simulink model "MSDR_v1"  (R2018a)
settings: Solver=ode23tb  StartTime=0.0  StopTime=50000  RelTol=1e-3
values from neighbouring files (symbols this model uses):
  a_f = -3.22E-5    (= -3.22e-05)    [MSDR_parameters.m]
  a_g = +2.35E-5    (= 2.35e-05)    [MSDR_parameters.m]
  beta = [0.000223, 0.001457, 0.001307, 0.002628, 0.000766, 0.000280]    [MSDR_parameters.m]
  beta_t = sum(beta)    [MSDR_parameters.m]
  Cp_s_shx = 1549.12e-6    (= 0.00154912)    [MSDR_parameters.m]
  Cst = 10    [MSDR_parameters.m]
  dLb = 0    [MSDR_parameters.m]
  dLs = 0    [MSDR_parameters.m]
  dLsc = 0    [MSDR_parameters.m]
  gamma_I = 5.1135e-2    (= 0.051135)    [MSDR_parameters.m]
  gamma_Xe = 1.1628e-2    (= 0.011628)    [MSDR_parameters.m]
  hA_fg = [h_fg*A_fg/2, h_fg*A_fg/2]    [MSDR_parameters.m]
  hA_p_phx1 = h_p_phx*A_p_phx    [MSDR_parameters.m]
  hA_p_phx2 = h_p_phx*A_p_phx    [MSDR_parameters.m]
  hA_p_phx3 = h_p_phx*A_p_phx    [MSDR_parameters.m]
  hA_p_phx4 = h_p_phx*A_p_phx    [MSDR_parameters.m]
  hA_p_phx5 = h_p_phx*A_p_phx    [MSDR_parameters.m]
  hA_p_phx6 = h_p_phx*A_p_phx    [MSDR_parameters.m]
  hA_p_shx1 = h_p_shx*A_p_shx    [MSDR_parameters.m]
  hA_p_shx2 = h_p_shx*A_p_shx    [MSDR_parameters.m]
  hA_p_shx3 = h_p_shx*A_p_shx    [MSDR_parameters.m]
  hA_p_shx4 = h_p_shx*A_p_shx    [MSDR_parameters.m]
  hA_p_shx5 = h_p_shx*A_p_shx    [MSDR_parameters.m]
  hA_p_shx6 = h_p_shx*A_p_shx    [MSDR_parameters.m]
  hA_s_phx1 = h_s_phx*A_s_phx    [MSDR_parameters.m]
  hA_s_phx2 = h_s_phx*A_s_phx    [MSDR_parameters.m]
  hA_s_phx3 = h_s_phx*A_s_phx    [MSDR_parameters.m]
  hA_s_phx4 = h_s_phx*A_s_phx    [MSDR_parameters.m]
  hA_s_phx5 = h_s_phx*A_s_phx    [MSDR_parameters.m]
  hA_s_phx6 = h_s_phx*A_s_phx    [MSDR_parameters.m]
  hA_s_shx1 = h_s_shx*A_s_shx    [MSDR_parameters.m]
  hA_s_shx2 = h_s_shx*A_s_shx    [MSDR_parameters.m]
  hA_s_shx3 = h_s_shx*A_s_shx    [MSDR_parameters.m]
  hA_s_shx4 = h_s_shx*A_s_shx    [MSDR_parameters.m]
  hA_s_shx5 = h_s_shx*A_s_shx    [MSDR_parameters.m]
  hA_s_shx6 = h_s_shx*A_s_shx    [MSDR_parameters.m]
  I_0 = gamma_I*Sig_f_msdr*phi_0/lam_I    (= 4.38204721773e+16)    [MSDR_parameters.m]
  Ifa = [0.25, 0.25]    [MSDR_parameters.m]
  Ifb = [0.25, 0.25]    [MSDR_parameters.m]
  Ig = [0.5, 0.5]    [MSDR_parameters.m]
  J = 1e-6    (= 1e-06)    [MSDR_parameters.m]
  ka = [0.235, 0.235]    [MSDR_parameters.m]
  kb = [0.235, 0.235]    [MSDR_parameters.m]
  kc = 5    [MSDR_parameters.m]
  kga = [0.015, 0.015]    [MSDR_parameters.m]
  kgb = [0.015, 0.015]    [MSDR_parameters.m]
  L = 8.5344    [MSDR_parameters.m]
  Lam = 2.400E-04    (= 0.00024)    [MSDR_parameters.m]
  lam = [0.0124, 0.0305, 0.111, 0.301, 1.14, 3.01]    [MSDR_parameters.m]
  lam_bubl = 2.0e-2    (= 0.02)    [MSDR_parameters.m]
  lam_I = 2.875e-5    (= 2.875e-05)    [MSDR_parameters.m]
  lam_Xe = 2.0916e-5    (= 2.0916e-05)    [MSDR_parameters.m]
  m_3m = W_3*2    (= 8618.207327)    [MSDR_parameters.m]
  m_fm = W_f*2    (= 9978.96)    [MSDR_parameters.m]
  m_sb = 1717    [MSDR_parameters.m]
  mb_cpb = 2.689619410657651e+00    (= 2.68961941066)    [MSDR_parameters.m]
  mcp_fa = mfa*Cp_f    [MSDR_parameters.m]
  mcp_fb = mfb*Cp_f    [MSDR_parameters.m]
  mcp_g = mg*Cp_g    [MSDR_parameters.m]
  mcp_p_phx1 = Cp_p_phx*mp_phx1    [MSDR_parameters.m]
  mcp_p_phx2 = Cp_p_phx*mp_phx2    [MSDR_parameters.m]
  mcp_p_phx3 = Cp_p_phx*mp_phx3    [MSDR_parameters.m]
  mcp_p_phx4 = Cp_p_phx*mp_phx4    [MSDR_parameters.m]
  mcp_p_phx5 = Cp_p_phx*mp_phx5    [MSDR_parameters.m]
  mcp_p_phx6 = Cp_p_phx*mp_phx6    [MSDR_parameters.m]
  mcp_p_shx1 = Cp_p_shx*mp_shx1    [MSDR_parameters.m]
  mcp_p_shx2 = Cp_p_shx*mp_shx2    [MSDR_parameters.m]
  mcp_p_shx3 = Cp_p_shx*mp_shx3    [MSDR_parameters.m]
  mcp_p_shx4 = Cp_p_shx*mp_shx4    [MSDR_parameters.m]
  mcp_p_shx5 = Cp_p_shx*mp_shx5    [MSDR_parameters.m]
  mcp_p_shx6 = Cp_p_shx*mp_shx6    [MSDR_parameters.m]
  mcp_s_phx1 = Cp_s_phx*ms_phx1    [MSDR_parameters.m]
  mcp_s_phx2 = Cp_s_phx*ms_phx2    [MSDR_parameters.m]
  mcp_s_phx3 = Cp_s_phx*ms_phx3    [MSDR_parameters.m]
  mcp_s_phx4 = Cp_s_phx*ms_phx4    [MSDR_parameters.m]
  mcp_s_phx5 = Cp_s_phx*ms_phx5    [MSDR_parameters.m]
  mcp_s_phx6 = Cp_s_phx*ms_phx6    [MSDR_parameters.m]
  mcp_s_shx1 = Cp_s_shx*ms_shx1    [MSDR_parameters.m]
  mcp_s_shx2 = Cp_s_shx*ms_shx1    [MSDR_parameters.m]
  mcp_s_shx3 = Cp_s_shx*ms_shx1    [MSDR_parameters.m]
  mcp_s_shx4 = Cp_s_shx*ms_shx1    [MSDR_parameters.m]
  mcp_s_shx5 = Cp_s_shx*ms_shx1    [MSDR_parameters.m]
  mcp_s_shx6 = Cp_s_shx*ms_shx1    [MSDR_parameters.m]
  mcp_t_phx1 = Cp_t_phx*mt_phx1    [MSDR_parameters.m]
  mcp_t_phx2 = Cp_t_phx*mt_phx2    [MSDR_parameters.m]
  mcp_t_phx3 = Cp_t_phx*mt_phx3    [MSDR_parameters.m]
  mcp_t_phx4 = Cp_t_phx*mt_phx4    [MSDR_parameters.m]
  mcp_t_phx5 = Cp_t_phx*mt_phx5    [MSDR_parameters.m]
  mcp_t_phx6 = Cp_t_phx*mt_phx6    [MSDR_parameters.m]
  mcp_t_shx1 = Cp_t_phx*mt_shx1    [MSDR_parameters.m]
  mcp_t_shx2 = Cp_t_phx*mt_shx2    [MSDR_parameters.m]
  mcp_t_shx3 = Cp_t_phx*mt_shx3    [MSDR_parameters.m]
  mcp_t_shx4 = Cp_t_phx*mt_shx4    [MSDR_parameters.m]
  mcp_t_shx5 = Cp_t_phx*mt_shx5    [MSDR_parameters.m]
  mcp_t_shx6 = Cp_t_phx*mt_shx6    [MSDR_parameters.m]
  mfa = [mass_fn, mass_fn]    [MSDR_parameters.m]
  mfb = [mass_fn, mass_fn]    [MSDR_parameters.m]
  mp_phx1 = [494.7, 494.7, 494.7, 494.7]    [MSDR_parameters.m]
  mp_phx2 = [494.7, 494.7, 494.7, 494.7]    [MSDR_parameters.m]
  mp_phx3 = [494.7, 494.7, 494.7, 494.7]    [MSDR_parameters.m]
  mp_phx4 = [494.7, 494.7, 494.7, 494.7]    [MSDR_parameters.m]
  mp_phx5 = [494.7, 494.7, 494.7, 494.7]    [MSDR_parameters.m]
  mp_phx6 = [494.7, 494.7, 494.7, 494.7]    [MSDR_parameters.m]
  mp_phxm = (Wp_phx1 + Wp_phx2)*1    (= 1663.16)    [MSDR_parameters.m]
  mp_shx1 = [429.3, 429.3, 429.3, 429.3]    [MSDR_parameters.m]
  mp_shx2 = [429.3, 429.3, 429.3, 429.3]    [MSDR_parameters.m]
  mp_shx3 = [429.3, 429.3, 429.3, 429.3]    [MSDR_parameters.m]
  mp_shx4 = [429.3, 429.3, 429.3, 429.3]    [MSDR_parameters.m]
  mp_shx5 = [429.3, 429.3, 429.3, 429.3]    [MSDR_parameters.m]
  mp_shx6 = [429.3, 429.3, 429.3, 429.3]    [MSDR_parameters.m]
  mp_shxm = (Wp_shx1 + Wp_shx2)*1    (= 932.38)    [MSDR_parameters.m]
  ms_phx1 = [1152.5, 1152.5, 1152.5, 1152.5]    [MSDR_parameters.m]
  ms_phx2 = [1152.5, 1152.5, 1152.5, 1152.5]    [MSDR_parameters.m]
  ms_phx3 = [1152.5, 1152.5, 1152.5, 1152.5]    [MSDR_parameters.m]
  ms_phx4 = [1152.5, 1152.5, 1152.5, 1152.5]    [MSDR_parameters.m]
  ms_phx5 = [1152.5, 1152.5, 1152.5, 1152.5]    [MSDR_parameters.m]
  ms_phx6 = [1152.5, 1152.5, 1152.5, 1152.5]    [MSDR_parameters.m]
  ms_phxm = (Ws_phx1 + Ws_phx2)*1    (= 932.38)    [MSDR_parameters.m]
  ms_shx1 = [1861.5, 1861.5, 1861.5, 1861.5]    [MSDR_parameters.m]
  ms_shx2 = [1861.5, 1861.5, 1861.5, 1861.5]    [MSDR_parameters.m]
  ... (+104 more)
undefined symbols (not defined in the file or in its folder): Ak2, As, C0, Cpp, Cps, Cpsc, Cpw, Dit, Dot, hA_p_thx1, hA_p_thx2, hA_p_thx3, hA_s_thx1, hA_s_thx2, hA_s_thx3, hc0, hfg, hfw0, HFW1, hfw10, HFW2, hpw, Hr, hr0, hwb, hws, hwsc, K3, KBHP, KBLP, Lsc, mcp_p_thx1, mcp_p_thx2, mcp_p_thx3, mcp_s_thx1, mcp_s_thx2, mcp_s_thx3, mcp_t_thx1, mcp_t_thx2, mcp_t_thx3, mp_thx1, mp_thx2, mp_thx3, ms_thx1, ms_thx2, ms_thx3, Mstm, nuf, Pp2, Pp3, Pp4, Pp5
libraries: simulink x20, aerolibconvert2 x2
(part 6 of 7)

== system MSDR_v1/HEAT EXCHANGERS/HEAT EXCHANGER LOOP 5/SHX3 HEAT TRANSFER ==
  PRIMARY FLUID INLET TEMPERATURE : Inport
  SECONDARY FLUID INLET TEMPERATURE : Inport  Port=2
  PRIMARY FLOW FRACTION : Inport  Port=3
  PRIMARY HEAT TRANSFER FRACTION : Inport  Port=4
  SECONDARY FLOW FRACTION : Inport  Port=5
  SECONDARY HEAT TRANSFER FRACTION : Inport  Port=6
  Mux : Mux  Inputs=16
      settings: DisplayOption=signals
  To Workspace : ToWorkspace  VariableName=shx3_ht  SampleTime=-1
  Tp1_shx3 : Integrator  InitialCondition=T0_p_shx3(1)
  Tp2_shx3 : Integrator  InitialCondition=T0_p_shx3(2)
  "Tp3_shx3 " : Integrator  InitialCondition=T0_p_shx3(3)
  Tp4_shx3 : Integrator  InitialCondition=T0_p_shx3(4)
  Ts1_shx3 : Integrator  InitialCondition=T0_s_shx3(1)
  Ts2_shx3 : Integrator  InitialCondition=T0_s_shx3(2)
  Ts3_shx3 : Integrator  InitialCondition=T0_s_shx3(3)
  Ts4_shx3 : Integrator  InitialCondition=T0_s_shx3(4)
  Tt1_shx3 : Integrator  InitialCondition=T0_t_shx3(1)
  Tt2_shx3 : Integrator  InitialCondition=T0_t_shx3(2)
  d(Tp1_shx3)/dt : Fcn  Expr=(u[13]*Wp_shx3/mp_shx3(1))*(u[1] - u[3]) + (u[14]*hA_p_shx3(1)/mcp_p_shx3(1))*(u[7] - u[3])
  d(Tp2_shx3)/dt : Fcn  Expr=(u[13]*Wp_shx3/mp_shx3(2))*(u[3] - u[4]) + (u[14]*hA_p_shx3(2)/mcp_p_shx3(2))*(u[7] - u[3])
  d(Tp3_shx3)/dt : Fcn  Expr=(u[13]*Wp_shx3/mp_shx3(3))*(u[4] - u[5]) + (u[14]*hA_p_shx3(3)/mcp_p_shx3(3))*(u[8] - u[5])
  d(Tp4_shx3)/dt : Fcn  Expr=(u[13]*Wp_shx3/mp_shx3(4))*(u[5] - u[6]) + (u[14]*hA_p_shx3(4)/mcp_p_shx3(4))*(u[8] - u[5])
  d(Ts1_shx3)/dt : Fcn  Expr=(u[15]*Ws_shx3/ms_shx3(1))*(u[2] - u[9]) + (u[16]*hA_s_shx3(1)/mcp_s_shx3(1))*(u[8] - u[9])
  d(Ts2_shx3)/dt : Fcn  Expr=(u[15]*Ws_shx3/ms_shx3(2))*(u[9] - u[10]) + (u[16]*hA_s_shx3(2)/mcp_s_shx3(2))*(u[8] - u[9])
  d(Ts3_shx3)/dt : Fcn  Expr=(u[15]*Ws_shx3/ms_shx3(3))*(u[10] - u[11]) + (u[16]*hA_s_shx3(3)/mcp_s_shx3(3))*(u[7] - u[11])
  d(Ts4_shx3)/dt : Fcn  Expr=(u[15]*Ws_shx3/ms_shx3(4))*(u[11] - u[12]) + (u[16]*hA_s_shx3(4)/mcp_s_shx3(4))*(u[7] - u[11])
  d(Tt1_shx3)/dt : Fcn  Expr=(u[14]*(hA_p_shx3(1) + hA_p_shx3(2))/mcp_t_shx3(1))*(u[3] - u[7]) + (u[16]*(hA_s_shx3(1) + hA_s_shx3(2))/mcp_t_shx3(1))*(u[11] - u[7])
  d(Tt2_shx3)/dt : Fcn  Expr=(u[14]*(hA_p_shx4(3) + hA_p_shx4(4))/mcp_t_shx4(2))*(u[5] - u[8]) + (u[16]*(hA_s_shx4(3) + hA_s_shx4(4))/mcp_t_shx4(2))*(u[9] - u[8])
  SHX3 TEMPERATURES : Outport
  wires:
  Ts1_shx3/1 -> Mux/9
  Ts2_shx3/1 -> Mux/10
  d(Ts2_shx3)/dt/1 -> Ts2_shx3/1
  d(Tp4_shx3)/dt/1 -> Tp4_shx3/1
  Tt1_shx3/1 -> Mux/7
  d(Tp2_shx3)/dt/1 -> Tp2_shx3/1
  Tp4_shx3/1 -> Mux/6
  d(Tt2_shx3)/dt/1 -> Tt2_shx3/1
  SECONDARY FLUID INLET TEMPERATURE/1 -> Mux/2
  Tt2_shx3/1 -> Mux/8
  Mux/1 -> To Workspace/1, SHX3 TEMPERATURES/1, d(Ts4_shx3)/dt/1, d(Ts3_shx3)/dt/1, d(Ts2_shx3)/dt/1, d(Ts1_shx3)/dt/1, d(Tt2_shx3)/dt/1, d(Tt1_shx3)/dt/1, d(Tp4_shx3)/dt/1, d(Tp3_shx3)/dt/1, d(Tp2_shx3)/dt/1, d(Tp1_shx3)/dt/1
  d(Tp1_shx3)/dt/1 -> Tp1_shx3/1
  d(Ts4_shx3)/dt/1 -> Ts4_shx3/1
  Tp1_shx3/1 -> Mux/3
  d(Ts1_shx3)/dt/1 -> Ts1_shx3/1
  d(Ts3_shx3)/dt/1 -> Ts3_shx3/1
  Ts3_shx3/1 -> Mux/11
  Ts4_shx3/1 -> Mux/12
  "Tp3_shx3 "/1 -> Mux/5
  d(Tp3_shx3)/dt/1 -> "Tp3_shx3 "/1
  Tp2_shx3/1 -> Mux/4
  d(Tt1_shx3)/dt/1 -> Tt1_shx3/1
  PRIMARY FLUID INLET TEMPERATURE/1 -> Mux/1
  PRIMARY FLOW FRACTION/1 -> Mux/13
  PRIMARY HEAT TRANSFER FRACTION/1 -> Mux/14
  SECONDARY FLOW FRACTION/1 -> Mux/15
  SECONDARY HEAT TRANSFER FRACTION/1 -> Mux/16

== system MSDR_v1/HEAT EXCHANGERS/HEAT EXCHANGER LOOP 5/SHX3 MATERIAL TRANSPORT ==
  SHX3 TEMPERATURES : Inport
  wires:
  SHX3 TEMPERATURES/1 -> ?

== system MSDR_v1/HEAT EXCHANGERS/HEAT EXCHANGER LOOP 5/SHX4 HEAT TRANSFER ==
  PRIMARY FLUID INLET TEMPERATURE : Inport
  SECONDARY FLUID INLET TEMPERATURE : Inport  Port=2
  PRIMARY FLOW FRACTION : Inport  Port=3
  PRIMARY HEAT TRANSFER FRACTION : Inport  Port=4
  SECONDARY FLOW FRACTION : Inport  Port=5
  SECONDARY HEAT TRANSFER FRACTION : Inport  Port=6
  Mux : Mux  Inputs=16
      settings: DisplayOption=signals
  To Workspace : ToWorkspace  VariableName=shx4_ht  SampleTime=-1
  Tp1_shx4 : Integrator  InitialCondition=T0_p_shx4(1)
  Tp2_shx4 : Integrator  InitialCondition=T0_p_shx4(2)
  "Tp3_shx4 " : Integrator  InitialCondition=T0_p_shx4(3)
  Tp4_shx4 : Integrator  InitialCondition=T0_p_shx4(4)
  Ts1_shx4 : Integrator  InitialCondition=T0_s_shx4(1)
  Ts2_shx4 : Integrator  InitialCondition=T0_s_shx4(2)
  Ts3_shx4 : Integrator  InitialCondition=T0_s_shx4(3)
  Ts4_shx4 : Integrator  InitialCondition=T0_s_shx4(4)
  Tt1_shx4 : Integrator  InitialCondition=T0_t_shx4(1)
  Tt2_shx4 : Integrator  InitialCondition=T0_t_shx4(2)
  d(Tp1_shx4)/dt : Fcn  Expr=(u[13]*Wp_shx4/mp_shx4(1))*(u[1] - u[3]) + (u[14]*hA_p_shx4(1)/mcp_p_shx4(1))*(u[7] - u[3])
  d(Tp2_shx4)/dt : Fcn  Expr=(u[13]*Wp_shx4/mp_shx4(2))*(u[3] - u[4]) + (u[14]*hA_p_shx4(2)/mcp_p_shx4(2))*(u[7] - u[3])
  d(Tp3_shx4)/dt : Fcn  Expr=(u[13]*Wp_shx4/mp_shx4(3))*(u[4] - u[5]) + (u[14]*hA_p_shx4(3)/mcp_p_shx4(3))*(u[8] - u[5])
  d(Tp4_shx4)/dt : Fcn  Expr=(u[13]*Wp_shx4/mp_shx4(4))*(u[5] - u[6]) + (u[14]*hA_p_shx4(4)/mcp_p_shx4(4))*(u[8] - u[5])
  d(Ts1_shx4)/dt : Fcn  Expr=(u[15]*Ws_shx4/ms_shx4(1))*(u[2] - u[9]) + (u[16]*hA_s_shx4(1)/mcp_s_shx4(1))*(u[8] - u[9])
  d(Ts2_shx4)/dt : Fcn  Expr=(u[15]*Ws_shx4/ms_shx4(2))*(u[9] - u[10]) + (u[16]*hA_s_shx4(2)/mcp_s_shx4(2))*(u[8] - u[9])
  d(Ts3_shx4)/dt : Fcn  Expr=(u[15]*Ws_shx4/ms_shx4(3))*(u[10] - u[11]) + (u[16]*hA_s_shx4(3)/mcp_s_shx4(3))*(u[7] - u[11])
  d(Ts4_shx4)/dt : Fcn  Expr=(u[15]*Ws_shx4/ms_shx4(4))*(u[11] - u[12]) + (u[16]*hA_s_shx4(4)/mcp_s_shx4(4))*(u[7] - u[11])
  d(Tt1_shx4)/dt : Fcn  Expr=(u[14]*(hA_p_shx4(1) + hA_p_shx4(2))/mcp_t_shx4(1))*(u[3] - u[7]) + (u[16]*(hA_s_shx4(1) + hA_s_shx4(2))/mcp_t_shx4(1))*(u[11] - u[7])
  d(Tt2_shx4)/dt : Fcn  Expr=(u[14]*(hA_p_shx4(3) + hA_p_shx4(4))/mcp_t_shx4(2))*(u[5] - u[8]) + (u[16]*(hA_s_shx4(3) + hA_s_shx4(4))/mcp_t_shx4(2))*(u[9] - u[8])
  SHX4 TEMPERATURES : Outport
  wires:
  Ts1_shx4/1 -> Mux/9
  Ts2_shx4/1 -> Mux/10
  d(Ts2_shx4)/dt/1 -> Ts2_shx4/1
  d(Tp4_shx4)/dt/1 -> Tp4_shx4/1
  Tt1_shx4/1 -> Mux/7
  d(Tp2_shx4)/dt/1 -> Tp2_shx4/1
  Tp4_shx4/1 -> Mux/6
  d(Tt2_shx4)/dt/1 -> Tt2_shx4/1
  SECONDARY FLUID INLET TEMPERATURE/1 -> Mux/2
  Tt2_shx4/1 -> Mux/8
  Mux/1 -> To Workspace/1, SHX4 TEMPERATURES/1, d(Ts4_shx4)/dt/1, d(Ts3_shx4)/dt/1, d(Ts2_shx4)/dt/1, d(Ts1_shx4)/dt/1, d(Tt2_shx4)/dt/1, d(Tt1_shx4)/dt/1, d(Tp4_shx4)/dt/1, d(Tp3_shx4)/dt/1, d(Tp2_shx4)/dt/1, d(Tp1_shx4)/dt/1
  d(Tp1_shx4)/dt/1 -> Tp1_shx4/1
  d(Ts4_shx4)/dt/1 -> Ts4_shx4/1
  Tp1_shx4/1 -> Mux/3
  d(Ts1_shx4)/dt/1 -> Ts1_shx4/1
  d(Ts3_shx4)/dt/1 -> Ts3_shx4/1
  Ts3_shx4/1 -> Mux/11
  Ts4_shx4/1 -> Mux/12
  "Tp3_shx4 "/1 -> Mux/5
  d(Tp3_shx4)/dt/1 -> "Tp3_shx4 "/1
  Tp2_shx4/1 -> Mux/4
  d(Tt1_shx4)/dt/1 -> Tt1_shx4/1
  PRIMARY FLUID INLET TEMPERATURE/1 -> Mux/1
  PRIMARY FLOW FRACTION/1 -> Mux/13
  PRIMARY HEAT TRANSFER FRACTION/1 -> Mux/14
  SECONDARY FLOW FRACTION/1 -> Mux/15
  SECONDARY HEAT TRANSFER FRACTION/1 -> Mux/16

== system MSDR_v1/HEAT EXCHANGERS/HEAT EXCHANGER LOOP 5/SHX4 MATERIAL TRANSPORT ==
  SHX4 TEMPERATURES : Inport
  wires:
  SHX4 TEMPERATURES/1 -> ?

== system MSDR_v1/HEAT EXCHANGERS/HEAT EXCHANGER LOOP 5/THX2 HEAT TRANSFER ==
  PRIMARY FLUID INLET TEMPERATURE : Inport
  SECONDARY FLUID INLET TEMPERATURE : Inport  Port=2
  PRIMARY FLOW FRACTION : Inport  Port=3
  PRIMARY HEAT TRANSFER FRACTION : Inport  Port=4
  SECONDARY FLOW FRACTION : Inport  Port=5
  SECONDARY HEAT TRANSFER FRACTION : Inport  Port=6
  Mux : Mux  Inputs=16
      settings: DisplayOption=signals
  To Workspace : ToWorkspace  VariableName=thx2_ht  SampleTime=-1
  Tp1_thx2 : Integrator  InitialCondition=T0_p_thx2(1)
  Tp2_thx2 : Integrator  InitialCondition=T0_p_thx2(2)
  "Tp3_thx2 " : Integrator  InitialCondition=T0_p_thx2(3)
  Tp4_thx2 : Integrator  InitialCondition=T0_p_thx2(4)
  Ts1_thx2 : Integrator  InitialCondition=T0_s_thx2(1)
  Ts2_thx2 : Integrator  InitialCondition=T0_s_thx2(2)
  Ts3_thx2 : Integrator  InitialCondition=T0_s_thx2(3)
  Ts4_thx2 : Integrator  InitialCondition=T0_s_thx2(4)
  Tt1_thx2 : Integrator  InitialCondition=T0_t_thx2(1)
  Tt2_thx2 : Integrator  InitialCondition=T0_t_thx2(2)
  d(Tp1_thx2)/dt : Fcn  Expr=(u[13]*Wp_thx2/mp_thx2(1))*(u[1] - u[3]) + (u[14]*hA_p_thx2(1)/mcp_p_thx2(1))*(u[7] - u[3])
  d(Tp2_thx2)/dt : Fcn  Expr=(u[13]*Wp_thx2/mp_thx2(2))*(u[3] - u[4]) + (u[14]*hA_p_thx2(2)/mcp_p_thx2(2))*(u[7] - u[3])
  d(Tp3_thx2)/dt : Fcn  Expr=(u[13]*Wp_thx2/mp_thx2(3))*(u[4] - u[5]) + (u14]*hA_p_thx2(3)/mcp_p_thx2(3))*(u[8] - u[5])
  d(Tp4_thx2)/dt : Fcn  Expr=(u[13]*Wp_thx2/mp_thx2(4))*(u[5] - u[6]) + (u[14]*hA_p_thx2(4)/mcp_p_thx2(4))*(u[8] - u[5])
  d(Ts1_thx2)/dt : Fcn  Expr=(u[15]*Ws_thx2/ms_thx2(1))*(u[2] - u[9]) + (u[16]*hA_s_thx2(1)/mcp_s_thx2(1))*(u[8] - u[9])
  d(Ts2_thx2)/dt : Fcn  Expr=(u[15]*Ws_thx2/ms_thx2(2))*(u[9] - u[10]) + (u[16]*hA_s_thx2(2)/mcp_s_thx2(2))*(u[8] - u[9])
  d(Ts3_thx2)/dt : Fcn  Expr=(u[15]*Ws_thx2/ms_thx2(3))*(u[10] - u[11]) + (u[16]*hA_s_thx2(3)/mcp_s_thx2(3))*(u[7] - u[11])
  d(Ts4_thx2)/dt : Fcn  Expr=(u[15]*Ws_thx2/ms_thx2(4))*(u[11] - u[12]) + (u[16]*hA_s_thx2(4)/mcp_s_thx2(4))*(u[7] - u[11])
  d(Tt1_thx2)/dt : Fcn  Expr=(u[14]*(hA_p_thx2(1) + hA_p_thx2(2))/mcp_t_thx2(1))*(u[3] - u[7]) + (u[16]*(hA_s_thx2(1) + hA_s_thx2(2))/mcp_t_thx2(1))*(u[11] - u[7])
  d(Tt2_thx2)/dt : Fcn  Expr=(u[14]*(hA_p_thx2(3) + hA_p_thx2(4))/mcp_t_thx2(2))*(u[5] - u[8]) + (u[16]*(hA_s_thx2(3) + hA_s_thx2(4))/mcp_t_thx2(2))*(u[9] - u[8])
  THX2 TEMPERATURES : Outport
  wires:
  Ts1_thx2/1 -> Mux/9
  Ts2_thx2/1 -> Mux/10
  d(Ts2_thx2)/dt/1 -> Ts2_thx2/1
  d(Tp4_thx2)/dt/1 -> Tp4_thx2/1
  Tt1_thx2/1 -> Mux/7
  d(Tp2_thx2)/dt/1 -> Tp2_thx2/1
  Tp4_thx2/1 -> Mux/6
  d(Tt2_thx2)/dt/1 -> Tt2_thx2/1
  SECONDARY FLUID INLET TEMPERATURE/1 -> Mux/2
  Tt2_thx2/1 -> Mux/8
  Mux/1 -> To Workspace/1, THX2 TEMPERATURES/1, d(Ts4_thx2)/dt/1, d(Ts3_thx2)/dt/1, d(Ts2_thx2)/dt/1, d(Ts1_thx2)/dt/1, d(Tt2_thx2)/dt/1, d(Tt1_thx2)/dt/1, d(Tp4_thx2)/dt/1, d(Tp3_thx2)/dt/1, d(Tp2_thx2)/dt/1, d(Tp1_thx2)/dt/1
  d(Tp1_thx2)/dt/1 -> Tp1_thx2/1
  d(Ts4_thx2)/dt/1 -> Ts4_thx2/1
  Tp1_thx2/1 -> Mux/3
  d(Ts1_thx2)/dt/1 -> Ts1_thx2/1
  d(Ts3_thx2)/dt/1 -> Ts3_thx2/1
  Ts3_thx2/1 -> Mux/11
  Ts4_thx2/1 -> Mux/12
  "Tp3_thx2 "/1 -> Mux/5
  d(Tp3_thx2)/dt/1 -> "Tp3_thx2 "/1
  Tp2_thx2/1 -> Mux/4
  d(Tt1_thx2)/dt/1 -> Tt1_thx2/1
  PRIMARY FLUID INLET TEMPERATURE/1 -> Mux/1
  PRIMARY FLOW FRACTION/1 -> Mux/13
  PRIMARY HEAT TRANSFER FRACTION/1 -> Mux/14
  SECONDARY FLOW FRACTION/1 -> Mux/15
  SECONDARY HEAT TRANSFER FRACTION/1 -> Mux/16

== system MSDR_v1/HEAT EXCHANGERS/HEAT EXCHANGER LOOP 5/THX2 MATERIAL TRANSPORT ==
  THX2 TEMPERATURES : Inport
  wires:
  THX2 TEMPERATURES/1 -> ?

== system MSDR_v1/HEAT EXCHANGERS/HEAT EXCHANGER LOOP 6/BOILER & REHEATER ==
  Coolant Inlet Temp : Inport
  Power Demand (Frac) : Inport  Port=2
  Fcn : Fcn  Commented=on  Expr=u[1] - u[2]*250/((Ws_shx1 + Ws_shx2)*Cp_s_shx)
  Integrator : Integrator  InitialCondition=400
  Mux : Mux  Inputs=3
      settings: DisplayOption=signals
  To Workspace : ToWorkspace  VariableName=msdr_br_mux3  SampleTime=-1
  ddt_t_b = 1/tau_b*(t_bin-t_b)-p_b/mb_cpb : Fcn  Expr=W_sb*(u(1)-u(3))/m_sb - u(2)/mb_cpb
  Coolant Exit Temp : Outport
  wires:
  Coolant Inlet Temp/1 -> Mux/1
  Mux/1 -> ddt_t_b = 1/tau_b*(t_bin-t_b)-p_b/mb_cpb/1, To Workspace/1
  Power Demand (Frac)/1 -> Mux/2
  Integrator/1 -> Coolant Exit Temp/1, Mux/3
  ddt_t_b = 1/tau_b*(t_bin-t_b)-p_b/mb_cpb/1 -> Integrator/1

== system MSDR_v1/HEAT EXCHANGERS/HEAT EXCHANGER LOOP 6/Fractional Power Demand (fractional) ==
  Add : Sum
  Constant : Constant
  Saturation : Saturate  UpperLimit=1  LowerLimit=0.2
  Saturation1 : Saturate  UpperLimit=.8  LowerLimit=0
  Slider : Subsystem  DialogController=hmiCreateDDGDialog  IsWebBlock=on  mask(MWDashboardBlock){webBlockId=9afe0574-93b5-4d2b-9630-def9aae4c12d, webBlockType=slider, ShowInLibBrowser=on, ShowInitialText=on, HMISrcModelName=MSDR_v1}
      mask prompts: webBlockId "WebBlock Id"; webBlockType "WebBlock Type"; HMISrcModelName "Source Model"
      mask help: SimulinkHMI:dialogs:SliderDialogDesc
      mask Help: helpview([docroot '/mapfiles/simulink.map'], 'hmi_slider')
      mask Display:
      | if strcmp(get_param(bdroot(gcb),'BlockDiagramType'), 'library')
      |     image([(matlabroot) '/toolbox/simulink/hmi/icons/Slider.png']);
      | end
  down 1%/min : simulink/Sources/Ramp  slope=-0.01/60  start=2500  InitialOutput=1
  up 1%/min1 : simulink/Sources/Ramp  slope=0.01/60  start=2500+3600+5000  InitialOutput=0
  Power Demand(frac) : Outport
  wires:
  down 1%/min/1 -> Saturation/1
  Saturation/1 -> Add/1
  up 1%/min1/1 -> Saturation1/1
  Saturation1/1 -> Add/2
  Constant/1 -> Power Demand(frac)/1

== system MSDR_v1/HEAT EXCHANGERS/HEAT EXCHANGER LOOP 6/PHX PRIM MIXING ==
  Tp_phx5 : Inport
  Tp_phx6 : Inport  Port=2
  p_flow_frac : Inport  Port=3
  Fcn : Fcn  Expr=u[3]*Wp_phx5/mp_phxm*(u[1]-u[4]) + u[3]*Wp_phx6/mp_phxm*(u[2]-u[4])
  Integrator : Integrator  InitialCondition=Tf_in
  Mux : Mux
  Tp_phx_mix : Outport
  wires:
  Tp_phx5/1 -> Mux/1
  Tp_phx6/1 -> Mux/2
  Mux/1 -> Fcn/1
  p_flow_frac/1 -> Mux/3
  Fcn/1 -> Integrator/1
  Integrator/1 -> Tp_phx_mix/1, Mux/4

== system MSDR_v1/HEAT EXCHANGERS/HEAT EXCHANGER LOOP 6/PHX SEC MIXING ==
  Ts_phx5 : Inport
  Ts_phx6 : Inport  Port=2
  s_flow_frac : Inport  Port=3
  Fcn : Fcn  Expr=u[3]*Ws_phx5/ms_phxm*(u[1]-u[4]) + u[3]*Ws_phx6/ms_phxm*(u[2]-u[4])
  Integrator : Integrator  InitialCondition=T0_s_phx1(4)
  Mux : Mux
  Ts_phx_mix : Outport
  wires:
  Ts_phx5/1 -> Mux/1
  Ts_phx6/1 -> Mux/2
  Mux/1 -> Fcn/1
  s_flow_frac/1 -> Mux/3
  Fcn/1 -> Integrator/1
  Integrator/1 -> Ts_phx_mix/1, Mux/4

== system MSDR_v1/HEAT EXCHANGERS/HEAT EXCHANGER LOOP 6/PHX//SHX PUMP ==
  1-D Lookup Table : Lookup_n-D  NumberOfTableDimensions=1  BreakpointsForDimension1=xdat  Table=ydat  InternalRulePriority=Speed  RndMeth=Simplest  InputSameDT=on
  Clock : Clock
  Fcn : Fcn  Expr=exp((1/tau_p)*u)
  Final convection flow rate : Constant  Value=therm_conv
  Scope : Scope
  Subtract : Sum  Inputs=-+
  Switch : Switch  Criteria=u2 > Threshold
  Transport Delay : TransportDelay  DelayTime=10000000  InitialOutput=1
  FLOW FRACTION : Outport
  HEAT TRANSFER FRACTION : Outport  Port=2
  wires:
  Transport Delay/1 -> 1-D Lookup Table/1, Scope/1, FLOW FRACTION/1
  Clock/1 -> Fcn/1
  Switch/1 -> Transport Delay/1
  Fcn/1 -> Subtract/1, Switch/1
  Final convection flow rate/1 -> Subtract/2, Switch/3
  Subtract/1 -> Switch/2
  1-D Lookup Table/1 -> HEAT TRANSFER FRACTION/1

== system MSDR_v1/HEAT EXCHANGERS/HEAT EXCHANGER LOOP 6/PHX5 HEAT TRANSFER ==
  PRIMARY FLUID INLET TEMPERATURE : Inport
  SECONDARY FLUID INLET TEMPERATURE : Inport  Port=2
  PRIMARY FLOW FRACTION : Inport  Port=3
  PRIMARY HEAT TRANSFER FRACTION : Inport  Port=4
  SECONDARY FLOW FRACTION : Inport  Port=5
  SECONDARY HEAT TRANSFER FRACTION : Inport  Port=6
  Mux : Mux  Inputs=16
      settings: DisplayOption=signals
  To Workspace : ToWorkspace  VariableName=phx5_ht  SampleTime=-1
  Tp1_phx5 : Integrator  InitialCondition=T0_p_phx5(1)
  Tp2_phx5 : Integrator  InitialCondition=T0_p_phx5(2)
  "Tp3_phx5 " : Integrator  InitialCondition=T0_p_phx5(3)
  Tp4_phx5 : Integrator  InitialCondition=T0_p_phx5(4)
  Ts1_phx5 : Integrator  InitialCondition=T0_s_phx5(1)
  Ts2_phx5 : Integrator  InitialCondition=T0_s_phx5(2)
  Ts3_phx5 : Integrator  InitialCondition=T0_s_phx5(3)
  Ts4_phx5 : Integrator  InitialCondition=T0_s_phx5(4)
  Tt1_phx5 : Integrator  InitialCondition=T0_t_phx5(1)
  Tt2_phx5 : Integrator  InitialCondition=T0_t_phx5(2)
  d(Tp1_phx5)/dt : Fcn  Expr=(u[13]*Wp_phx5/mp_phx5(1))*(u[1] - u[3]) + (u[14]*hA_p_phx5(1)/mcp_p_phx5(1))*(u[7] - u[3])
  d(Tp2_phx5)/dt : Fcn  Expr=(u[13]*Wp_phx5/mp_phx5(2))*(u[3] - u[4]) + (u[14]*hA_p_phx5(2)/mcp_p_phx5(2))*(u[7] - u[3])
  d(Tp3_phx5)/dt : Fcn  Expr=(u[13]*Wp_phx5/mp_phx5(3))*(u[4] - u[5]) + (u[14]*hA_p_phx5(3)/mcp_p_phx5(3))*(u[8] - u[5])
  d(Tp4_phx5)/dt : Fcn  Expr=(u[13]*Wp_phx5/mp_phx5(4))*(u[5] - u[6]) + (u[14]*hA_p_phx5(4)/mcp_p_phx5(4))*(u[8] - u[5])
  d(Ts1_phx5)/dt : Fcn  Expr=(u[15]*Ws_phx5/ms_phx5(1))*(u[2] - u[9]) + (u[16]*hA_s_phx5(1)/mcp_s_phx5(1))*(u[8] - u[9])
  d(Ts2_phx5)/dt : Fcn  Expr=(u[15]*Ws_phx5/ms_phx5(2))*(u[9] - u[10]) + (u[16]*hA_s_phx5(2)/mcp_s_phx5(2))*(u[8] - u[9])
  d(Ts3_phx5)/dt : Fcn  Expr=(u[15]*Ws_phx5/ms_phx5(3))*(u[10] - u[11]) + (u[16]*hA_s_phx5(3)/mcp_s_phx5(3))*(u[7] - u[11])
  d(Ts4_phx5)/dt : Fcn  Expr=(u[15]*Ws_phx5/ms_phx5(4))*(u[11] - u[12]) + (u[16]*hA_s_phx5(4)/mcp_s_phx5(4))*(u[7] - u[11])
  d(Tt1_phx3)/dt : Fcn  Expr=(u[14]*(hA_p_phx5(1) + hA_p_phx5(2))/mcp_t_phx5(1))*(u[3] - u[7]) + (u[16]*(hA_s_phx5(1) + hA_s_phx5(2))/mcp_t_phx5(1))*(u[11] - u[7])
  d(Tt2_phx5)/dt : Fcn  Expr=(u[14]*(hA_p_phx5(3) + hA_p_phx5(4))/mcp_t_phx5(2))*(u[5] - u[8]) + (u[16]*(hA_s_phx5(3) + hA_s_phx5(4))/mcp_t_phx5(2))*(u[9] - u[8])
  PHX5 TEMPERATURES : Outport
  wires:
  Ts1_phx5/1 -> Mux/9
  Ts2_phx5/1 -> Mux/10
  d(Ts2_phx5)/dt/1 -> Ts2_phx5/1
  d(Tp4_phx5)/dt/1 -> Tp4_phx5/1
  Tt1_phx5/1 -> Mux/7
  d(Tp2_phx5)/dt/1 -> Tp2_phx5/1
  Tp4_phx5/1 -> Mux/6
  d(Tt2_phx5)/dt/1 -> Tt2_phx5/1
  SECONDARY FLUID INLET TEMPERATURE/1 -> Mux/2
  Tt2_phx5/1 -> Mux/8
  Mux/1 -> To Workspace/1, PHX5 TEMPERATURES/1, d(Ts4_phx5)/dt/1, d(Ts3_phx5)/dt/1, d(Ts1_phx5)/dt/1, d(Tt2_phx5)/dt/1, d(Tt1_phx3)/dt/1, d(Tp4_phx5)/dt/1, d(Tp3_phx5)/dt/1, d(Tp2_phx5)/dt/1, d(Tp1_phx5)/dt/1, d(Ts2_phx5)/dt/1
  d(Tp1_phx5)/dt/1 -> Tp1_phx5/1
  d(Ts4_phx5)/dt/1 -> Ts4_phx5/1
  Tp1_phx5/1 -> Mux/3
  d(Ts1_phx5)/dt/1 -> Ts1_phx5/1
  d(Ts3_phx5)/dt/1 -> Ts3_phx5/1
  Ts3_phx5/1 -> Mux/11
  Ts4_phx5/1 -> Mux/12
  "Tp3_phx5 "/1 -> Mux/5
  d(Tp3_phx5)/dt/1 -> "Tp3_phx5 "/1
  Tp2_phx5/1 -> Mux/4
  d(Tt1_phx3)/dt/1 -> Tt1_phx5/1
  PRIMARY FLUID INLET TEMPERATURE/1 -> Mux/1
  PRIMARY FLOW FRACTION/1 -> Mux/13
  PRIMARY HEAT TRANSFER FRACTION/1 -> Mux/14
  SECONDARY FLOW FRACTION/1 -> Mux/15
  SECONDARY HEAT TRANSFER FRACTION/1 -> Mux/16

== system MSDR_v1/HEAT EXCHANGERS/HEAT EXCHANGER LOOP 6/PHX5 MATERIAL TRANSPORT ==
  PHX5 TEMPERATURES : Inport
  wires:
  PHX5 TEMPERATURES/1 -> ?

== system MSDR_v1/HEAT EXCHANGERS/HEAT EXCHANGER LOOP 6/PHX6 HEAT TRANSFER ==
  PRIMARY FLUID INLET TEMPERATURE : Inport
  SECONDARY FLUID INLET TEMPERATURE : Inport  Port=2
  PRIMARY FLOW FRACTION : Inport  Port=3
  PRIMARY HEAT TRANSFER FRACTION : Inport  Port=4
  SECONDARY FLOW FRACTION : Inport  Port=5
  SECONDARY HEAT TRANSFER FRACTION : Inport  Port=6
  Mux : Mux  Inputs=16
      settings: DisplayOption=signals
  To Workspace : ToWorkspace  VariableName=phx6_ht  SampleTime=-1
  Tp1_phx6 : Integrator  InitialCondition=T0_p_phx6(1)
  Tp2_phx6 : Integrator  InitialCondition=T0_p_phx6(2)
  "Tp3_phx6 " : Integrator  InitialCondition=T0_p_phx6(3)
  Tp4_phx6 : Integrator  InitialCondition=T0_p_phx6(4)
  Ts1_phx6 : Integrator  InitialCondition=T0_s_phx6(1)
  Ts2_phx6 : Integrator  InitialCondition=T0_s_phx6(2)
  Ts3_phx6 : Integrator  InitialCondition=T0_s_phx6(3)
  Ts4_phx6 : Integrator  InitialCondition=T0_s_phx6(4)
  Tt1_phx6 : Integrator  InitialCondition=T0_t_phx6(1)
  Tt2_phx6 : Integrator  InitialCondition=T0_t_phx6(2)
  d(Tp1_phx6)/dt : Fcn  Expr=(u[13]*Wp_phx6/mp_phx6(1))*(u[1] - u[3]) + (u[14]*hA_p_phx6(1)/mcp_p_phx6(1))*(u[7] - u[3])
  d(Tp2_phx6)/dt : Fcn  Expr=(u[13]*Wp_phx6/mp_phx6(2))*(u[3] - u[4]) + (u[14]*hA_p_phx6(2)/mcp_p_phx6(2))*(u[7] - u[3])
  d(Tp3_phx6)/dt : Fcn  Expr=(u[13]*Wp_phx6/mp_phx6(3))*(u[4] - u[5]) + (u[14]*hA_p_phx6(3)/mcp_p_phx6(3))*(u[8] - u[5])
  d(Tp4_phx6)/dt : Fcn  Expr=(u[13]*Wp_phx6/mp_phx6(4))*(u[5] - u[6]) + (u[14]*hA_p_phx6(4)/mcp_p_phx6(4))*(u[8] - u[5])
  d(Ts1_phx6)/dt : Fcn  Expr=(u[15]*Ws_phx6/ms_phx6(1))*(u[2] - u[9]) + (u[16]*hA_s_phx6(1)/mcp_s_phx6(1))*(u[8] - u[9])
  d(Ts2_phx6)/dt : Fcn  Expr=(u[15]*Ws_phx6/ms_phx6(2))*(u[9] - u[10]) + (u[16]*hA_s_phx6(2)/mcp_s_phx6(2))*(u[8] - u[9])
  d(Ts3_phx6)/dt : Fcn  Expr=(u[15]*Ws_phx6/ms_phx6(3))*(u[10] - u[11]) + (u[16]*hA_s_phx6(3)/mcp_s_phx6(3))*(u[7] - u[11])
  d(Ts4_phx6)/dt : Fcn  Expr=(u[15]*Ws_phx6/ms_phx6(4))*(u[11] - u[12]) + (u[16]*hA_s_phx6(4)/mcp_s_phx6(4))*(u[7] - u[11])
  d(Tt1_phx6)/dt : Fcn  Expr=(u[14]*(hA_p_phx6(1) + hA_p_phx6(2))/mcp_t_phx6(1))*(u[3] - u[7]) + (u[16]*(hA_s_phx6(1) + hA_s_phx6(2))/mcp_t_phx6(1))*(u[11] - u[7])
  d(Tt2_phx6)/dt : Fcn  Expr=(u[14]*(hA_p_phx6(3) + hA_p_phx6(4))/mcp_t_phx6(2))*(u[5] - u[8]) + (u[16]*(hA_s_phx6(3) + hA_s_phx6(4))/mcp_t_phx6(2))*(u[9] - u[8])
  PHX6 TEMPERATURES : Outport
  wires:
  Ts1_phx6/1 -> Mux/9
  Ts2_phx6/1 -> Mux/10
  d(Ts2_phx6)/dt/1 -> Ts2_phx6/1
  d(Tp4_phx6)/dt/1 -> Tp4_phx6/1
  Tt1_phx6/1 -> Mux/7
  d(Tp2_phx6)/dt/1 -> Tp2_phx6/1
  Tp4_phx6/1 -> Mux/6
  d(Tt2_phx6)/dt/1 -> Tt2_phx6/1
  SECONDARY FLUID INLET TEMPERATURE/1 -> Mux/2
  Tt2_phx6/1 -> Mux/8
  Mux/1 -> To Workspace/1, PHX6 TEMPERATURES/1, d(Ts4_phx6)/dt/1, d(Ts3_phx6)/dt/1, d(Ts1_phx6)/dt/1, d(Tt2_phx6)/dt/1, d(Tt1_phx6)/dt/1, d(Tp4_phx6)/dt/1, d(Tp3_phx6)/dt/1, d(Tp2_phx6)/dt/1, d(Tp1_phx6)/dt/1, d(Ts2_phx6)/dt/1
  d(Tp1_phx6)/dt/1 -> Tp1_phx6/1
  d(Ts4_phx6)/dt/1 -> Ts4_phx6/1
  Tp1_phx6/1 -> Mux/3
  d(Ts1_phx6)/dt/1 -> Ts1_phx6/1
  d(Ts3_phx6)/dt/1 -> Ts3_phx6/1
  Ts3_phx6/1 -> Mux/11
  Ts4_phx6/1 -> Mux/12
  "Tp3_phx6 "/1 -> Mux/5
  d(Tp3_phx6)/dt/1 -> "Tp3_phx6 "/1
  Tp2_phx6/1 -> Mux/4
  d(Tt1_phx6)/dt/1 -> Tt1_phx6/1
  PRIMARY FLUID INLET TEMPERATURE/1 -> Mux/1
  SECONDARY FLOW FRACTION/1 -> Mux/15
  PRIMARY HEAT TRANSFER FRACTION/1 -> Mux/14
  PRIMARY FLOW FRACTION/1 -> Mux/13
  SECONDARY HEAT TRANSFER FRACTION/1 -> Mux/16

== system MSDR_v1/HEAT EXCHANGERS/HEAT EXCHANGER LOOP 6/PHX6 MATERIAL TRANSPORT ==
  PHX6 TEMPERATURES : Inport
  wires:
  PHX6 TEMPERATURES/1 -> ?

== system MSDR_v1/HEAT EXCHANGERS/HEAT EXCHANGER LOOP 6/SHX PRIM MIXING ==
  Tp_shx5 : Inport
  Tp_shx6 : Inport  Port=2
  p_flow_frac : Inport  Port=3
  Fcn : Fcn  Expr=u[3]*Wp_shx5/mp_shxm*(u[1]-u[4]) + u[3]*Wp_shx6/mp_shxm*(u[2]-u[4])
  Integrator : Integrator  InitialCondition=T0_p_shx1(4)
  Mux : Mux
  Tp_shx_mix : Outport
  wires:
  Tp_shx5/1 -> Mux/1
  Tp_shx6/1 -> Mux/2
  Mux/1 -> Fcn/1
  p_flow_frac/1 -> Mux/3
  Fcn/1 -> Integrator/1
  Integrator/1 -> Tp_shx_mix/1, Mux/4

== system MSDR_v1/HEAT EXCHANGERS/HEAT EXCHANGER LOOP 6/SHX SEC MIXING ==
  Ts_shx5 : Inport
  Ts_shx6 : Inport  Port=2
  s_flow_frac : Inport  Port=3
  Fcn : Fcn  Expr=u[3]*Ws_shx5/ms_shxm*(u[1]-u[4]) + u[3]*Ws_shx6/ms_shxm*(u[2]-u[4])
  Integrator : Integrator  InitialCondition=T0_s_shx1(4)
  Mux : Mux
  Ts_shx_mix : Outport
  wires:
  Ts_shx5/1 -> Mux/1
  Ts_shx6/1 -> Mux/2
  Mux/1 -> Fcn/1
  s_flow_frac/1 -> Mux/3
  Fcn/1 -> Integrator/1
  Integrator/1 -> Ts_shx_mix/1, Mux/4

== system MSDR_v1/HEAT EXCHANGERS/HEAT EXCHANGER LOOP 6/SHX//THX PUMP ==
  1-D Lookup Table : Lookup_n-D  NumberOfTableDimensions=1  BreakpointsForDimension1=xdat  Table=ydat  InternalRulePriority=Speed  RndMeth=Simplest  InputSameDT=on
  Clock : Clock
  Fcn : Fcn  Expr=exp((1/tau_p)*u)
  Final convection flow rate : Constant  Value=therm_conv
  Scope : Scope
  Subtract : Sum  Inputs=-+
  Switch : Switch  Criteria=u2 > Threshold
  Transport Delay : TransportDelay  DelayTime=20000000  InitialOutput=1
  FLOW FRACTION : Outport
  HEAT TRANSFER FRACTION : Outport  Port=2
  wires:
  Transport Delay/1 -> 1-D Lookup Table/1, Scope/1, FLOW FRACTION/1
  Clock/1 -> Fcn/1
  Switch/1 -> Transport Delay/1
  Fcn/1 -> Subtract/1, Switch/1
  Final convection flow rate/1 -> Subtract/2, Switch/3
  Subtract/1 -> Switch/2
  1-D Lookup Table/1 -> HEAT TRANSFER FRACTION/1

== system MSDR_v1/HEAT EXCHANGERS/HEAT EXCHANGER LOOP 6/SHX5 HEAT TRANSFER ==
  PRIMARY FLUID INLET TEMPERATURE : Inport
  SECONDARY FLUID INLET TEMPERATURE : Inport  Port=2
  PRIMARY FLOW FRACTION : Inport  Port=3
  PRIMARY HEAT TRANSFER FRACTION : Inport  Port=4
  SECONDARY FLOW FRACTION : Inport  Port=5
  SECONDARY HEAT TRANSFER FRACTION : Inport  Port=6
  Mux : Mux  Inputs=16
      settings: DisplayOption=signals
  To Workspace : ToWorkspace  VariableName=shx5_ht  SampleTime=-1
  Tp1_shx5 : Integrator  InitialCondition=T0_p_shx3(1)
  Tp2_shx5 : Integrator  InitialCondition=T0_p_shx5(2)
  "Tp3_shx5 " : Integrator  InitialCondition=T0_p_shx5(3)
  Tp4_shx5 : Integrator  InitialCondition=T0_p_shx5(4)
  Ts1_shx5 : Integrator  InitialCondition=T0_s_shx5(1)
  Ts2_shx5 : Integrator  InitialCondition=T0_s_shx5(2)
  Ts3_shx5 : Integrator  InitialCondition=T0_s_shx5(3)
  Ts4_shx5 : Integrator  InitialCondition=T0_s_shx5(4)
  Tt1_shx5 : Integrator  InitialCondition=T0_t_shx5(1)
  Tt2_shx5 : Integrator  InitialCondition=T0_t_shx5(2)
  d(Tp1_shx5)/dt : Fcn  Expr=(u[13]*Wp_shx5/mp_shx5(1))*(u[1] - u[3]) + (u[14]*hA_p_shx5(1)/mcp_p_shx5(1))*(u[7] - u[3])
  d(Tp2_shx5)/dt : Fcn  Expr=(u[13]*Wp_shx5/mp_shx5(2))*(u[3] - u[4]) + (u[14]*hA_p_shx5(2)/mcp_p_shx5(2))*(u[7] - u[3])
  d(Tp3_shx5)/dt : Fcn  Expr=(u[13]*Wp_shx5/mp_shx5(3))*(u[4] - u[5]) + (u[14]*hA_p_shx5(3)/mcp_p_shx5(3))*(u[8] - u[5])
  d(Tp4_shx5)/dt : Fcn  Expr=(u[13]*Wp_shx5/mp_shx5(4))*(u[5] - u[6]) + (u[14]*hA_p_shx5(4)/mcp_p_shx5(4))*(u[8] - u[5])
  d(Ts1_shx5)/dt : Fcn  Expr=(u[15]*Ws_shx5/ms_shx5(1))*(u[2] - u[9]) + (u[16]*hA_s_shx5(1)/mcp_s_shx5(1))*(u[8] - u[9])
  d(Ts2_shx5)/dt : Fcn  Expr=(u[15]*Ws_shx5/ms_shx5(2))*(u[9] - u[10]) + (u[16]*hA_s_shx5(2)/mcp_s_shx5(2))*(u[8] - u[9])
  d(Ts3_shx5)/dt : Fcn  Expr=(u[15]*Ws_shx5/ms_shx5(3))*(u[10] - u[11]) + (u[16]*hA_s_shx5(3)/mcp_s_shx5(3))*(u[7] - u[11])
  d(Ts4_shx5)/dt : Fcn  Expr=(u[15]*Ws_shx5/ms_shx5(4))*(u[11] - u[12]) + (u[16]*hA_s_shx5(4)/mcp_s_shx5(4))*(u[7] - u[11])
  d(Tt1_shx5)/dt : Fcn  Expr=(u[14]*(hA_p_shx5(1) + hA_p_shx5(2))/mcp_t_shx5(1))*(u[3] - u[7]) + (u[16]*(hA_s_shx5(1) + hA_s_shx5(2))/mcp_t_shx5(1))*(u[11] - u[7])
  d(Tt2_shx5)/dt : Fcn  Expr=(u[14]*(hA_p_shx5(3) + hA_p_shx5(4))/mcp_t_shx5(2))*(u[5] - u[8]) + (u[16]*(hA_s_shx5(3) + hA_s_shx5(4))/mcp_t_shx5(2))*(u[9] - u[8])
  SHX5 TEMPERATURES : Outport
  wires:
  Ts1_shx5/1 -> Mux/9
  Ts2_shx5/1 -> Mux/10
  d(Ts2_shx5)/dt/1 -> Ts2_shx5/1
  d(Tp4_shx5)/dt/1 -> Tp4_shx5/1
  Tt1_shx5/1 -> Mux/7
  d(Tp2_shx5)/dt/1 -> Tp2_shx5/1
  Tp4_shx5/1 -> Mux/6
  d(Tt2_shx5)/dt/1 -> Tt2_shx5/1
  SECONDARY FLUID INLET TEMPERATURE/1 -> Mux/2
  Tt2_shx5/1 -> Mux/8
  Mux/1 -> To Workspace/1, SHX5 TEMPERATURES/1, d(Ts4_shx5)/dt/1, d(Ts3_shx5)/dt/1, d(Ts2_shx5)/dt/1, d(Ts1_shx5)/dt/1, d(Tt2_shx5)/dt/1, d(Tt1_shx5)/dt/1, d(Tp4_shx5)/dt/1, d(Tp3_shx5)/dt/1, d(Tp2_shx5)/dt/1, d(Tp1_shx5)/dt/1
  d(Tp1_shx5)/dt/1 -> Tp1_shx5/1
  d(Ts4_shx5)/dt/1 -> Ts4_shx5/1
  Tp1_shx5/1 -> Mux/3
  d(Ts1_shx5)/dt/1 -> Ts1_shx5/1
  d(Ts3_shx5)/dt/1 -> Ts3_shx5/1
  Ts3_shx5/1 -> Mux/11
  Ts4_shx5/1 -> Mux/12
  "Tp3_shx5 "/1 -> Mux/5
  d(Tp3_shx5)/dt/1 -> "Tp3_shx5 "/1
  Tp2_shx5/1 -> Mux/4
  d(Tt1_shx5)/dt/1 -> Tt1_shx5/1
  PRIMARY FLUID INLET TEMPERATURE/1 -> Mux/1
  SECONDARY FLOW FRACTION/1 -> Mux/15
  PRIMARY HEAT TRANSFER FRACTION/1 -> Mux/14
  PRIMARY FLOW FRACTION/1 -> Mux/13
  SECONDARY HEAT TRANSFER FRACTION/1 -> Mux/16

== system MSDR_v1/HEAT EXCHANGERS/HEAT EXCHANGER LOOP 6/SHX5 MATERIAL TRANSPORT ==
  SHX5 TEMPERATURES : Inport
  wires:
  SHX5 TEMPERATURES/1 -> ?

== system MSDR_v1/HEAT EXCHANGERS/HEAT EXCHANGER LOOP 6/SHX6 HEAT TRANSFER ==
  PRIMARY FLUID INLET TEMPERATURE : Inport
  SECONDARY FLUID INLET TEMPERATURE : Inport  Port=2
  PRIMARY FLOW FRACTION : Inport  Port=3
  PRIMARY HEAT TRANSFER FRACTION : Inport  Port=4
  SECONDARY FLOW FRACTION : Inport  Port=5
  SECONDARY HEAT TRANSFER FRACTION : Inport  Port=6
  Mux : Mux  Inputs=16
      settings: DisplayOption=signals
  To Workspace : ToWorkspace  VariableName=shx6_ht  SampleTime=-1
  Tp1_shx6 : Integrator  InitialCondition=T0_p_shx6(1)
  Tp2_shx6 : Integrator  InitialCondition=T0_p_shx6(2)
  "Tp3_shx6 " : Integrator  InitialCondition=T0_p_shx6(3)
  Tp4_shx6 : Integrator  InitialCondition=T0_p_shx6(4)
  Ts1_shx6 : Integrator  InitialCondition=T0_s_shx6(1)
  Ts2_shx6 : Integrator  InitialCondition=T0_s_shx6(2)
  Ts3_shx6 : Integrator  InitialCondition=T0_s_shx6(3)
  Ts4_shx6 : Integrator  InitialCondition=T0_s_shx6(4)
  Tt1_shx6 : Integrator  InitialCondition=T0_t_shx6(1)
  Tt2_shx6 : Integrator  InitialCondition=T0_t_shx6(2)
  d(Tp1_shx6)/dt : Fcn  Expr=(u[13]*Wp_shx6/mp_shx6(1))*(u[1] - u[3]) + (u[14]*hA_p_shx6(1)/mcp_p_shx6(1))*(u[7] - u[3])
  d(Tp2_shx6)/dt : Fcn  Expr=(u[13]*Wp_shx6/mp_shx6(2))*(u[3] - u[4]) + (u[14]*hA_p_shx6(2)/mcp_p_shx6(2))*(u[7] - u[3])
  d(Tp3_shx6)/dt : Fcn  Expr=(u[13]*Wp_shx6/mp_shx6(3))*(u[4] - u[5]) + (u[14]*hA_p_shx6(3)/mcp_p_shx6(3))*(u[8] - u[5])
  d(Tp4_shx6)/dt : Fcn  Expr=(u[13]*Wp_shx6/mp_shx6(4))*(u[5] - u[6]) + (u[14]*hA_p_shx6(4)/mcp_p_shx6(4))*(u[8] - u[5])
  d(Ts1_shx6)/dt : Fcn  Expr=(u[15]*Ws_shx6/ms_shx6(1))*(u[2] - u[9]) + (u[16]*hA_s_shx6(1)/mcp_s_shx6(1))*(u[8] - u[9])
  d(Ts2_shx6)/dt : Fcn  Expr=(u[15]*Ws_shx6/ms_shx6(2))*(u[9] - u[10]) + (u[16]*hA_s_shx6(2)/mcp_s_shx6(2))*(u[8] - u[9])
  d(Ts3_shx6)/dt : Fcn  Expr=(u[15]*Ws_shx6/ms_shx6(3))*(u[10] - u[11]) + (u[16]*hA_s_shx6(3)/mcp_s_shx6(3))*(u[7] - u[11])
  d(Ts4_shx4)/dt : Fcn  Expr=(u[15]*Ws_shx6/ms_shx6(4))*(u[11] - u[12]) + (u[16]*hA_s_shx6(4)/mcp_s_shx6(4))*(u[7] - u[11])
  d(Tt1_shx6)/dt : Fcn  Expr=(u[14]*(hA_p_shx6(1) + hA_p_shx6(2))/mcp_t_shx6(1))*(u[3] - u[7]) + (u[16]*(hA_s_shx6(1) + hA_s_shx6(2))/mcp_t_shx6(1))*(u[11] - u[7])
  d(Tt2_shx6)/dt : Fcn  Expr=(u[14]*(hA_p_shx6(3) + hA_p_shx6(4))/mcp_t_shx6(2))*(u[5] - u[8]) + (u[16]*(hA_s_shx6(3) + hA_s_shx6(4))/mcp_t_shx6(2))*(u[9] - u[8])
  SHX6 TEMPERATURES : Outport
  wires:
  Ts1_shx6/1 -> Mux/9
  Ts2_shx6/1 -> Mux/10
  d(Ts2_shx6)/dt/1 -> Ts2_shx6/1
  d(Tp4_shx6)/dt/1 -> Tp4_shx6/1
  Tt1_shx6/1 -> Mux/7
  d(Tp2_shx6)/dt/1 -> Tp2_shx6/1
  Tp4_shx6/1 -> Mux/6
  d(Tt2_shx6)/dt/1 -> Tt2_shx6/1
  SECONDARY FLUID INLET TEMPERATURE/1 -> Mux/2
  Tt2_shx6/1 -> Mux/8
  Mux/1 -> To Workspace/1, SHX6 TEMPERATURES/1, d(Ts4_shx4)/dt/1, d(Ts3_shx6)/dt/1, d(Ts2_shx6)/dt/1, d(Ts1_shx6)/dt/1, d(Tt2_shx6)/dt/1, d(Tt1_shx6)/dt/1, d(Tp4_shx6)/dt/1, d(Tp3_shx6)/dt/1, d(Tp2_shx6)/dt/1, d(Tp1_shx6)/dt/1
  d(Tp1_shx6)/dt/1 -> Tp1_shx6/1
  d(Ts4_shx4)/dt/1 -> Ts4_shx6/1
  Tp1_shx6/1 -> Mux/3
  d(Ts1_shx6)/dt/1 -> Ts1_shx6/1
  d(Ts3_shx6)/dt/1 -> Ts3_shx6/1
  Ts3_shx6/1 -> Mux/11
  Ts4_shx6/1 -> Mux/12
  "Tp3_shx6 "/1 -> Mux/5
  d(Tp3_shx6)/dt/1 -> "Tp3_shx6 "/1
  Tp2_shx6/1 -> Mux/4
  d(Tt1_shx6)/dt/1 -> Tt1_shx6/1
  PRIMARY FLUID INLET TEMPERATURE/1 -> Mux/1
  SECONDARY FLOW FRACTION/1 -> Mux/15
  PRIMARY HEAT TRANSFER FRACTION/1 -> Mux/14
  PRIMARY FLOW FRACTION/1 -> Mux/13
  SECONDARY HEAT TRANSFER FRACTION/1 -> Mux/16

== system MSDR_v1/HEAT EXCHANGERS/HEAT EXCHANGER LOOP 6/SHX6 MATERIAL TRANSPORT ==
  SHX6 TEMPERATURES : Inport
  wires:
  SHX6 TEMPERATURES/1 -> ?

== system MSDR_v1/HEAT EXCHANGERS/HEAT EXCHANGER LOOP 6/THX2 HEAT TRANSFER ==
  PRIMARY FLUID INLET TEMPERATURE : Inport
  SECONDARY FLUID INLET TEMPERATURE : Inport  Port=2
  PRIMARY FLOW FRACTION : Inport  Port=3
  PRIMARY HEAT TRANSFER FRACTION : Inport  Port=4
  SECONDARY FLOW FRACTION : Inport  Port=5
  SECONDARY HEAT TRANSFER FRACTION : Inport  Port=6
  Mux : Mux  Inputs=16
      settings: DisplayOption=signals
  To Workspace : ToWorkspace  VariableName=thx3_ht  SampleTime=-1
  Tp1_thx3 : Integrator  InitialCondition=T0_p_thx3(1)
  Tp2_thx3 : Integrator  InitialCondition=T0_p_thx3(2)
  "Tp3_thx3 " : Integrator  InitialCondition=T0_p_thx3(3)
  Tp4_thx3 : Integrator  InitialCondition=T0_p_thx3(4)
  Ts1_thx3 : Integrator  InitialCondition=T0_s_thx3(1)
  Ts2_thx3 : Integrator  InitialCondition=T0_s_thx3(2)
  Ts3_thx3 : Integrator  InitialCondition=T0_s_thx3(3)
  Ts4_thx3 : Integrator  InitialCondition=T0_s_thx3(4)
  Tt1_thx3 : Integrator  InitialCondition=T0_t_thx3(1)
  Tt2_thx3 : Integrator  InitialCondition=T0_t_thx3(2)
  d(Tp1_thx3)/dt : Fcn  Expr=(u[13]*Wp_thx3/mp_thx3(1))*(u[1] - u[3]) + (u[14]*hA_p_thx3(1)/mcp_p_thx3(1))*(u[7] - u[3])
  d(Tp2_thx3)/dt : Fcn  Expr=(u[13]*Wp_thx3/mp_thx3(2))*(u[3] - u[4]) + (u[14]*hA_p_thx3(2)/mcp_p_thx3(2))*(u[7] - u[3])
  d(Tp3_thx3)/dt : Fcn  Expr=(u[13]*Wp_thx3/mp_thx3(3))*(u[4] - u[5]) + (u[14]*hA_p_thx3(3)/mcp_p_thx3(3))*(u[8] - u[5])
  d(Tp4_thx3)/dt : Fcn  Expr=(u[13]*Wp_thx3/mp_thx3(4))*(u[5] - u[6]) + (u[14]*hA_p_thx3(4)/mcp_p_thx3(4))*(u[8] - u[5])
  d(Ts1_thx3)/dt : Fcn  Expr=(u[15]*Ws_thx3/ms_thx3(1))*(u[2] - u[9]) + (u[16]*hA_s_thx3(1)/mcp_s_thx3(1))*(u[8] - u[9])
  d(Ts2_thx3)/dt : Fcn  Expr=(u[15]*Ws_thx3/ms_thx3(2))*(u[9] - u[10]) + (u[16]*hA_s_thx3(2)/mcp_s_thx3(2))*(u[8] - u[9])
  d(Ts3_thx3)/dt : Fcn  Expr=(u[15]*Ws_thx3/ms_thx3(3))*(u[10] - u[11]) + (u[16]*hA_s_thx3(3)/mcp_s_thx3(3))*(u[7] - u[11])
  d(Ts4_thx3)/dt : Fcn  Expr=(u[15]*Ws_thx3/ms_thx3(4))*(u[11] - u[12]) + (u[16]*hA_s_thx3(4)/mcp_s_thx3(4))*(u[7] - u[11])
  d(Tt1_thx3)/dt : Fcn  Expr=(u[14]*(hA_p_thx3(1) + hA_p_thx3(2))/mcp_t_thx3(1))*(u[3] - u[7]) + (u[16]*(hA_s_thx3(1) + hA_s_thx3(2))/mcp_t_thx3(1))*(u[11] - u[7])
  d(Tt2_thx3)/dt : Fcn  Expr=(u[14]*(hA_p_thx3(3) + hA_p_thx3(4))/mcp_t_thx3(2))*(u[5] - u[8]) + (u[16]*(hA_s_thx3(3) + hA_s_thx3(4))/mcp_t_thx3(2))*(u[9] - u[8])
  THX3 TEMPERATURES : Outport
  wires:
  Ts1_thx3/1 -> Mux/9
  Ts2_thx3/1 -> Mux/10
  d(Ts2_thx3)/dt/1 -> Ts2_thx3/1
  d(Tp4_thx3)/dt/1 -> Tp4_thx3/1
  Tt1_thx3/1 -> Mux/7
  d(Tp2_thx3)/dt/1 -> Tp2_thx3/1
  Tp4_thx3/1 -> Mux/6
  d(Tt2_thx3)/dt/1 -> Tt2_thx3/1
  SECONDARY FLUID INLET TEMPERATURE/1 -> Mux/2
  Tt2_thx3/1 -> Mux/8
  Mux/1 -> To Workspace/1, THX3 TEMPERATURES/1, d(Ts4_thx3)/dt/1, d(Ts3_thx3)/dt/1, d(Ts2_thx3)/dt/1, d(Ts1_thx3)/dt/1, d(Tt2_thx3)/dt/1, d(Tt1_thx3)/dt/1, d(Tp4_thx3)/dt/1, d(Tp3_thx3)/dt/1, d(Tp2_thx3)/dt/1, d(Tp1_thx3)/dt/1
  d(Tp1_thx3)/dt/1 -> Tp1_thx3/1
  d(Ts4_thx3)/dt/1 -> Ts4_thx3/1
  Tp1_thx3/1 -> Mux/3
  d(Ts1_thx3)/dt/1 -> Ts1_thx3/1
  d(Ts3_thx3)/dt/1 -> Ts3_thx3/1
  Ts3_thx3/1 -> Mux/11
  Ts4_thx3/1 -> Mux/12
  "Tp3_thx3 "/1 -> Mux/5
  d(Tp3_thx3)/dt/1 -> "Tp3_thx3 "/1
  Tp2_thx3/1 -> Mux/4
  d(Tt1_thx3)/dt/1 -> Tt1_thx3/1
  PRIMARY FLUID INLET TEMPERATURE/1 -> Mux/1
  SECONDARY HEAT TRANSFER FRACTION/1 -> Mux/16
  PRIMARY FLOW FRACTION/1 -> Mux/13
  PRIMARY HEAT TRANSFER FRACTION/1 -> Mux/14
  SECONDARY FLOW FRACTION/1 -> Mux/15

== system MSDR_v1/HEAT EXCHANGERS/HEAT EXCHANGER LOOP 6/THX3 MATERIAL TRANSPORT ==
  THX3 TEMPERATURES : Inport
  wires:
  THX3 TEMPERATURES/1 -> ?

== system MSDR_v1/BALANCE OF PLANT/POWER/BOP/H.P. Turbine ==
  note: h2=hc-nhp(hc-h'2)
  note: ((u[6]-u[3])-u[2])/T_w2
  note: ((u[5]-u[9])/eta_hp_isen)+u[9]
  note: 1067+0.37*(PR-200)-0.0011*(PR-200)^2-0.1*(PC-1000)
  note: ((h'2-hc)/eta_hp_isen)+hc
  note: KBHP*u[6]
  note: KBHP*w2
  note: ((w2-wBHP)-w''2)*(1/T_w2)
  note: 1067+0.37*(u[8]/144-200)-0.0011*(u[8]/144-200)^2-0.1*(u[7]/144-1000)
  note: u[9]-0.3*(u[9]-u[5])
  W2 : Inport
  hc : Inport  Port=2
  PC : Inport  Port=3
  PR : Inport  Port=4
  Display1 : Display
  Display20 : Display
  IC5 : InitialCondition  Value=1131
  Mux1 : Mux  Inputs=9
      settings: DisplayOption=signals
  dw''2/dt : Fcn  Expr=((u[6]-u[3])-u[2])/T_w2
  h'2 : Fcn  Expr=1067+0.37*(u[8]/144-200)-0.0011*(u[8]/144-200)^2-0.1*(u[7]/144-1000)
  h2_calc : Fcn  Expr=u[9]-0.3*(u[9]-u[5])
  output : ToWorkspace  VariableName=hpt  SampleTime=-1
  w''2 : Integrator  InitialCondition=w2_hpout
  wBHP : Fcn  Expr=KBHP*u[6]
  W2'' : Outport
  WBHP : Outport  Port=2
  h2 : Outport  Port=3
  wires:
  dw''2/dt/1 -> w''2/1, Mux1/1
  w''2/1 -> W2''/1, Mux1/2
  W2/1 -> Mux1/6
  hc/1 -> Mux1/9
  PC/1 -> Mux1/7
  PR/1 -> Mux1/8
  h2_calc/1 -> Display1/1, h2/1, Mux1/4
  wBHP/1 -> WBHP/1, Mux1/3
  h'2/1 -> Display20/1, Mux1/5
  Mux1/1 -> output/1, IC5/1, wBHP/1, dw''2/dt/1, h'2/1
  IC5/1 -> h2_calc/1

== system MSDR_v1/BALANCE OF PLANT/POWER/BOP/Heater 1 ==
  note: (u[3]/TH1*u[7])+(u[11]-u[2])/TH1
  note: Tco
  note: u(9)+u(13)+u(12)
  note: Wco'+WBLP+W1HP
  note: HFW1*(w1HP+wBLP)
  note: (QH1/(TH1*wfw))+(h0-h1fw)/TH1
  note: HFW1*(u[12]+u[13])
  WBLP : Inport
  Tco : Inport  Port=2
  Wco' : Inport  Port=3
  W1HP : Inport  Port=4
  h0 : Inport  Port=5
  1/Wfw1 : Math  Operator=reciprocal  SaturateOnIntegerOverflow=on
  Fcn : Fcn  Expr=u(10)
  Init1 : InitialCondition  Value=1/Wfw
  Init2 : InitialCondition  Value=Wfw
  Mux1 : Mux  Inputs=13
      settings: DisplayOption=signals
  QH1 : Fcn  Expr=HFW1*(u[12]+u[13])
  Scope{,1..7} (8 alike) : Scope
  Tci : Constant  VectorParams1D=off
  Tci1 : Constant  VectorParams1D=off
  Wfw_calc : Fcn  Expr=u(9)+u(13)+u(12)
  dh1fw/dt : Fcn  Expr=(u[3]/TH1*u[7])+(u[11]-u[2])/TH1
  h1fw_calc : Integrator  InitialCondition=hfw10
  ho : Lookup  InputValues=[162.18,170.00,182.81,193.16,211.95,227.92,240.03]  Table=[130.18 138.02 150.86 161.25 180.16 196.27 208.52]  RndMeth=Nearest  SaturateOnIntegerOverflow=on
  output : ToWorkspace  VariableName=fha  SampleTime=-1
  Wfw_out : Outport
  h1fw : Outport  Port=2
  wires:
  dh1fw/dt/1 -> Mux1/1, h1fw_calc/1, Scope4/1
  h1fw_calc/1 -> Mux1/2, Scope2/1, h1fw/1
  WBLP/1 -> Mux1/13, Scope7/1
  W1HP/1 -> Scope6/1, Mux1/12
  QH1/1 -> Scope1/1, Mux1/3
  Fcn/1 -> ho/1
  ho/1 -> Mux1/8, Scope/1
  1/Wfw1/1 -> Init1/1
  Tco/1 -> Mux1/10
  Wco'/1 -> Scope5/1, Mux1/9
  Wfw_calc/1 -> Init2/1
  Tci1/1 -> Mux1/5
  Tci/1 -> Mux1/4
  Mux1/1 -> Fcn/1, Wfw_calc/1, dh1fw/dt/1, QH1/1, output/1
  Init1/1 -> Scope3/1, Mux1/7
  Init2/1 -> Mux1/6, Wfw_out/1, 1/Wfw1/1
  h0/1 -> Mux1/11

== system MSDR_v1/BALANCE OF PLANT/POWER/BOP/Heater 2 ==
  note: 0.95484181*u[2] + 38.33195608
  note: ((w2-w'2)/TH2P)+((w1PR-w1HP)/TH2P)
  note: HFW2*(wBHP+wMS+w1PR)
  note: (QH2/(TH2*wfw))+(h1fw-hfw)/TH2
  note: (u[3]/TH2*u[13])+(u[7]-u[2])/TH2
  note: HFW2*(u[8]+u[9]+u[10])
  note: ((u[11]-u[12])/TH2P)+((u[10]-u[5])/TH2P)
  WBHP : Inport
  WM.S. : Inport  Port=2
  W1PR : Inport  Port=3
  w'2 : Inport  Port=4
  Wfw : Inport  Port=5
  h1fw : Inport  Port=6
  w2 : Inport  Port=7
  1/Wfw : Math  Operator=reciprocal  SaturateOnIntegerOverflow=on
  Init4 : InitialCondition  Value=Wfw
  Mux1 : Mux  Inputs=13
      settings: DisplayOption=signals
  QH2 : Fcn  Expr=HFW2*(u[8]+u[9]+u[10])
  Scope{,1..5} (6 alike) : Scope
  Tfw_calc : Fcn  Expr=0.95484181*u[2] + 38.33195608
  dhfw/dt : Fcn  Expr=(u[3]/TH2*u[13])+(u[7]-u[2])/TH2
  dw1HP/dt : Fcn  Expr=((u[11]-u[12])/TH2P)+((u[10]-u[5])/TH2P)
  hfw_ : Integrator  InitialCondition=hfw0
  output : ToWorkspace  VariableName=fhb  SampleTime=-1
  w1HP : Integrator  InitialCondition=whp10
  Tfw : Outport
  Wfw_out : Outport  Port=2
  W1HP : Outport  Port=3
  wires:
  dhfw/dt/1 -> Scope4/1, Mux1/1, hfw_/1
  hfw_/1 -> Scope/1, Mux1/2
  dw1HP/dt/1 -> Mux1/4, w1HP/1
  w1HP/1 -> W1HP/1, Scope2/1, Mux1/5
  h1fw/1 -> Scope5/1, Mux1/7
  WBHP/1 -> Mux1/8
  WM.S./1 -> Mux1/9
  W1PR/1 -> Mux1/10
  w2/1 -> Mux1/11
  w'2/1 -> Mux1/12
  1/Wfw/1 -> Mux1/13
  Wfw/1 -> Init4/1
  QH2/1 -> Scope1/1, Mux1/3
  Mux1/1 -> output/1, dw1HP/dt/1, QH2/1, dhfw/dt/1, Tfw_calc/1
  Init4/1 -> 1/Wfw/1, Wfw_out/1
  Tfw_calc/1 -> Scope3/1, Mux1/6, Tfw/1

== system MSDR_v1/BALANCE OF PLANT/POWER/BOP/I.P. and L.P. Turbine ==
  note: u[5]-0.3*(u[5]-898)
  note: (u(4)-u(3)-u(2))/t_w3
  note: (w3-wBLP-w3')/t_w3
  note: KBLP*u[4]
  note: KBLP*w3
  W3 : Inport
  hR : Inport  Port=2
  Mux1 : Mux  Inputs=6
      settings: DisplayOption=signals
  dw'3/dt : Fcn  Expr=(u(4)-u(3)-u(2))/T_w3
  h4 : Fcn  Expr=u[5]-0.3*(u[5]-898)
  output : ToWorkspace  VariableName=lpt  SampleTime=-1
  scope{1..3,6} (4 alike) : Scope
  w'3 : Integrator  InitialCondition=w3_lpout
  wBLP : Fcn  Expr=KBLP*u[4]
  W'3 : Outport
  WBLP : Outport  Port=2
  h4_out : Outport  Port=3
  wires:
  dw'3/dt/1 -> w'3/1, scope2/1, Mux1/1
  w'3/1 -> scope3/1, W'3/1, Mux1/2
  W3/1 -> scope6/1, Mux1/4
  Mux1/1 -> output/1, h4/1, dw'3/dt/1, wBLP/1
  wBLP/1 -> WBLP/1, Mux1/3, scope1/1
  hR/1 -> Mux1/5
  h4/1 -> Mux1/6, h4_out/1

== system MSDR_v1/BALANCE OF PLANT/POWER/BOP/Moisture Separator ==
  note: (u[7]-u[8])-u[2]
  note: ((h2-hf)/hfg)*w''2
  note: (w2-KBHP*w2)-w2'
  note: ((u[6]-u[3])*u[4])*u[5]
  hfg : Inport
  hf : Inport  Port=2
  w2 : Inport  Port=3
  w2'' : Inport  Port=4
  h2 : Inport  Port=5
  Wbhp : Inport  Port=6
  1/hfg : Math  Operator=reciprocal  SaturateOnIntegerOverflow=on
  Display{1..3,24} (4 alike) : Display
  Mux1 : Mux  Inputs=8
      settings: DisplayOption=signals
  output : ToWorkspace  VariableName=msr  SampleTime=-1
  w'2 : Fcn  Expr=((u[6]-u[3])*u[4])*u[5]
  w'2_90% : Fcn  Expr=u[5]*0.9
  wms : Fcn  Expr=(u[7]-u[8])-u[2]
  wms_10% : Fcn  Expr=u[5]*0.1
  w2'_out : Outport
  wms_out : Outport  Port=2
  wires:
  Mux1/1 -> output/1, w'2_90%/1, wms_10%/1, wms/1, w'2/1
  w2''/1 -> Mux1/5
  h2/1 -> Mux1/6
  hfg/1 -> 1/hfg/1
  w2/1 -> Mux1/7
  1/hfg/1 -> Mux1/4
  hf/1 -> Mux1/3
  Wbhp/1 -> Mux1/8
  w'2/1 -> Display24/1
  w'2_90%/1 -> Display3/1, w2'_out/1, Mux1/2
  wms/1 -> Display1/1
  wms_10%/1 -> Display2/1, wms_out/1, Mux1/1
